simulink model "moving_average_smoother"  (R2021a)
settings: Solver=FixedStepAuto  StartTime=0.0  StopTime=10.0  RelTol=1e-3
undefined symbols (not defined in the file): enable_smoother
libraries: dspstat3 x3
settings Model: Creator=esl  LastModifiedBy=esl

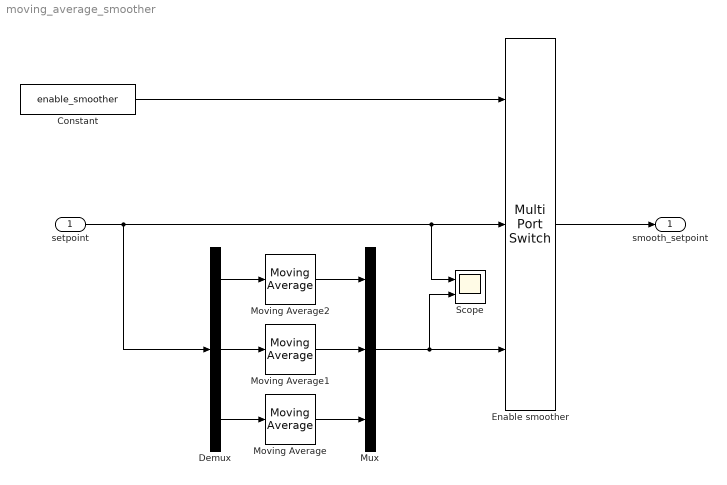
== system moving_average_smoother ==
  setpoint : Inport
  Constant : Constant  Value=enable_smoother
  Demux : Demux  Outputs=3
  Enable smoother : MultiPortSwitch  DataPortOrder=Zero-based contiguous  Inputs=2  zeroidx=on
  Moving Average : dspstat3/Moving Average  Method=Exponential weighting  ForgettingFactorPort=off  SpecifyWindowLength=on  WindowLength=4  ForgettingFactor=moving_ave_exp  SimulateUsing=Code generation
  Moving Average1 : dspstat3/Moving Average  Method=Exponential weighting  ForgettingFactorPort=off  SpecifyWindowLength=on  WindowLength=4  ForgettingFactor=moving_ave_exp  SimulateUsing=Code generation
  Moving Average2 : dspstat3/Moving Average  Method=Exponential weighting  ForgettingFactorPort=off  SpecifyWindowLength=on  WindowLength=4  ForgettingFactor=moving_ave_exp  SimulateUsing=Code generation
  Mux : Mux  Inputs=3
  Scope : Scope  NumInputPorts=2
  smooth_setpoint : Outport
  wires:
  Demux/3 -> Moving Average/1
  Moving Average1/1 -> Mux/2
  Moving Average2/1 -> Mux/1
  Moving Average/1 -> Mux/3
  Demux/1 -> Moving Average2/1
  Demux/2 -> Moving Average1/1
  Enable smoother/1 -> smooth_setpoint/1
  setpoint/1 -> Demux/1, Enable smoother/2, Scope/1
  Constant/1 -> Enable smoother/1
  Mux/1 -> Scope/2, Enable smoother/3
